simulink model "alu"  (R2022b)
settings: Solver=VariableStepAuto  StartTime=0.0  StopTime=10.0  RelTol=1e-3
settings Model: Creator=F1  LastModifiedBy=Namratha
settings SolverCC: AlgebraicLoopSolver=TrustRegion
settings DebuggingCC: UnconnectedInputMsg=warning  UnconnectedOutputMsg=warning  UnconnectedLineMsg=warning  SFMachineParentedDataDiag=warning
settings ModelReferenceCC: EnableRefExpFcnMdlSchedulingChecks=on

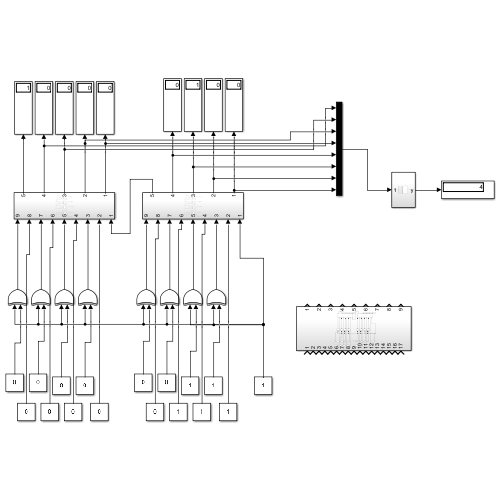
[thumbnail: Simulink's stored preview of the top-level diagram]
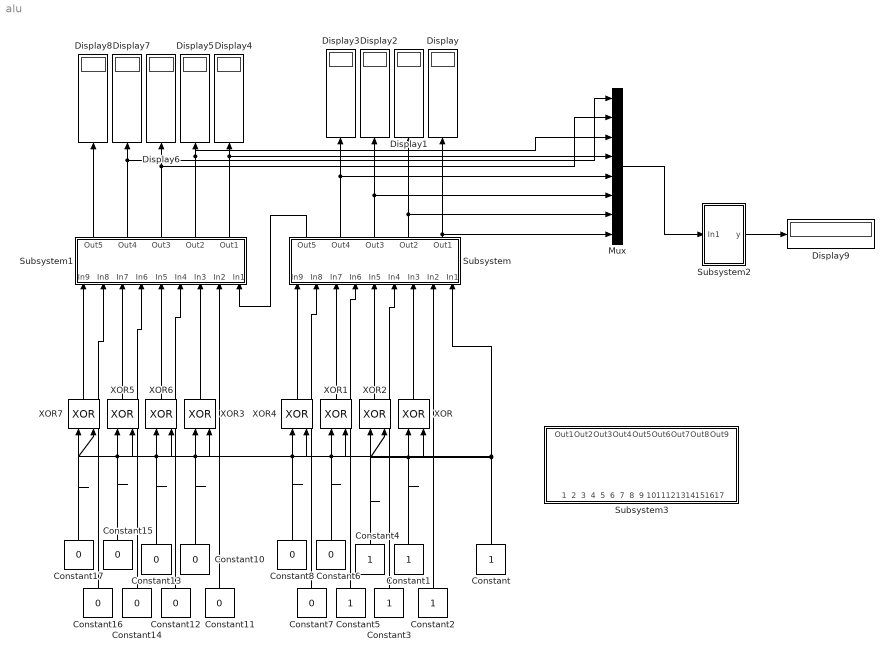
== system alu ==
  Constant{,1..5} (6 alike) : Constant
  Constant{6..8,10..17} (11 alike) : Constant  Value=0
  Display{,1..9} (10 alike) : Display
  Mux : Mux  Inputs=8
  Subsystem : Subsystem
  Subsystem1 : Subsystem
  Subsystem2 : Subsystem
  Subsystem3 : Subsystem
  XOR{,1..7} (8 alike) : Logic  Operator=XOR  IconShape=distinctive  AllPortsSameDT=off  OutDataTypeStr=boolean
  wires:
  XOR/1 -> Subsystem/3(In3)
  XOR2/1 -> Subsystem/5(In5)
  XOR1/1 -> Subsystem/7(In7)
  XOR4/1 -> Subsystem/9(In9)
  Constant1/1 -> XOR/2
  Constant2/1 -> Subsystem/2(In2)
  Constant3/1 -> Subsystem/4(In4)
  Constant4/1 -> XOR2/2
  Constant5/1 -> Subsystem/6(In6)
  Constant6/1 -> XOR1/2
  Constant7/1 -> Subsystem/8(In8)
  Constant8/1 -> XOR4/2
  Constant12/1 -> Subsystem1/4(In4)
  Constant15/1 -> XOR5/2
  XOR3/1 -> Subsystem1/3(In3)
  Constant/1 -> XOR2/1, XOR/1, XOR5/1, XOR7/1, XOR6/1, XOR3/1, XOR4/1, XOR1/1, Subsystem/1(In1)
  Constant13/1 -> XOR6/2
  Constant11/1 -> Subsystem1/2(In2)
  Constant16/1 -> Subsystem1/8(In8)
  Constant10/1 -> XOR3/2
  XOR7/1 -> Subsystem1/9(In9)
  XOR6/1 -> Subsystem1/5(In5)
  Constant17/1 -> XOR7/2
  XOR5/1 -> Subsystem1/7(In7)
  Constant14/1 -> Subsystem1/6(In6)
  Subsystem/5(Out5) -> Subsystem1/1(In1)
  Subsystem/1(Out1) -> Display/1, Mux/8
  Subsystem/2(Out2) -> Display1/1, Mux/7
  Subsystem/3(Out3) -> Display2/1, Mux/6
  Subsystem/4(Out4) -> Display3/1, Mux/5
  Subsystem1/1(Out1) -> Mux/4, Display4/1
  Subsystem1/2(Out2) -> Mux/3, Display5/1
  Subsystem1/3(Out3) -> Display6/1, Mux/2
  Subsystem1/4(Out4) -> Display7/1, Mux/1
  Subsystem1/5(Out5) -> Display8/1
  Mux/1 -> Subsystem2/1(In1)
  Subsystem2/1(y) -> Display9/1

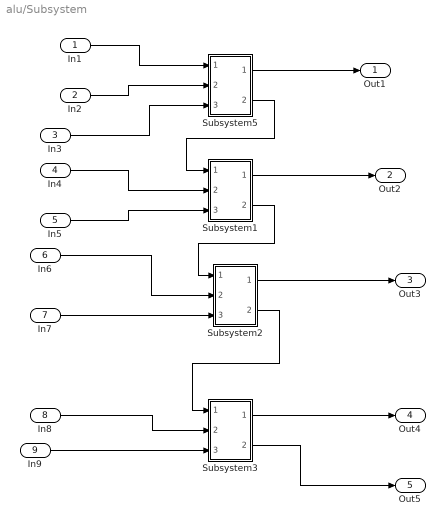
== system alu/Subsystem ==
  In1 : Inport
  In2 : Inport  Port=2
  In3 : Inport  Port=3
  In4 : Inport  Port=4
  In5 : Inport  Port=5
  In6 : Inport  Port=6
  In7 : Inport  Port=7
  In8 : Inport  Port=8
  In9 : Inport  Port=9
  Subsystem1 : Subsystem
  Subsystem2 : Subsystem
  Subsystem3 : Subsystem
  Subsystem5 : Subsystem
  Out1 : Outport
  Out2 : Outport  Port=2
  Out3 : Outport  Port=3
  Out4 : Outport  Port=4
  Out5 : Outport  Port=5
  wires:
  Subsystem2/2(Out2) -> Subsystem3/1(In1)
  In8/1 -> Subsystem3/2(In2)
  Subsystem5/2(Out2) -> Subsystem1/1(In1)
  Subsystem2/1(Out1) -> Out3/1
  Subsystem1/2(Out2) -> Subsystem2/1(In1)
  In6/1 -> Subsystem2/2(In2)
  In7/1 -> Subsystem2/3(In3)
  In4/1 -> Subsystem1/2(In2)
  Subsystem3/1(Out1) -> Out4/1
  In9/1 -> Subsystem3/3(In3)
  In2/1 -> Subsystem5/2(In2)
  In3/1 -> Subsystem5/3(In3)
  In1/1 -> Subsystem5/1(In1)
  Subsystem5/1(Out1) -> Out1/1
  Subsystem3/2(Out2) -> Out5/1
  Subsystem1/1(Out1) -> Out2/1
  In5/1 -> Subsystem1/3(In3)

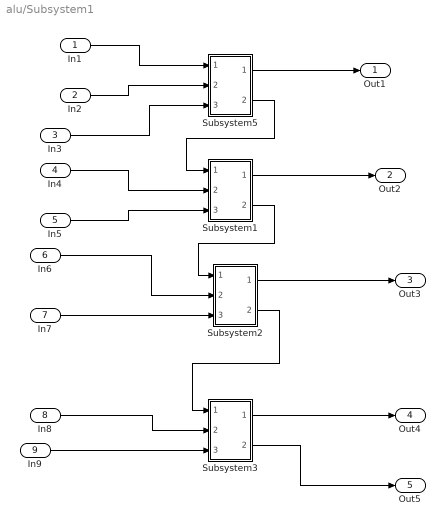
== system alu/Subsystem1 ==
  In1 : Inport
  In2 : Inport  Port=2
  In3 : Inport  Port=3
  In4 : Inport  Port=4
  In5 : Inport  Port=5
  In6 : Inport  Port=6
  In7 : Inport  Port=7
  In8 : Inport  Port=8
  In9 : Inport  Port=9
  Subsystem1 : Subsystem
  Subsystem2 : Subsystem
  Subsystem3 : Subsystem
  Subsystem5 : Subsystem
  Out1 : Outport
  Out2 : Outport  Port=2
  Out3 : Outport  Port=3
  Out4 : Outport  Port=4
  Out5 : Outport  Port=5
  wires:
  Subsystem2/2(Out2) -> Subsystem3/1(In1)
  In8/1 -> Subsystem3/2(In2)
  Subsystem5/2(Out2) -> Subsystem1/1(In1)
  Subsystem2/1(Out1) -> Out3/1
  Subsystem1/2(Out2) -> Subsystem2/1(In1)
  In6/1 -> Subsystem2/2(In2)
  In7/1 -> Subsystem2/3(In3)
  In4/1 -> Subsystem1/2(In2)
  Subsystem3/1(Out1) -> Out4/1
  In9/1 -> Subsystem3/3(In3)
  In2/1 -> Subsystem5/2(In2)
  In3/1 -> Subsystem5/3(In3)
  In1/1 -> Subsystem5/1(In1)
  Subsystem5/1(Out1) -> Out1/1
  Subsystem3/2(Out2) -> Out5/1
  Subsystem1/1(Out1) -> Out2/1
  In5/1 -> Subsystem1/3(In3)

== system alu/Subsystem2 ==
  In1 : Inport
  Demux : Demux  Outputs=8
  MATLAB Function : MATLAB Function  TreatAsAtomicUnit=on
  y : Outport
  wires:
  Demux/8 -> MATLAB Function/8(b0)
  Demux/2 -> MATLAB Function/2(b6)
  MATLAB Function/1(y) -> y/1
  Demux/7 -> MATLAB Function/7(b1)
  Demux/4 -> MATLAB Function/4(b4)
  Demux/6 -> MATLAB Function/6(b2)
  Demux/3 -> MATLAB Function/3(b5)
  Demux/1 -> MATLAB Function/1(b7)
  Demux/5 -> MATLAB Function/5(b3)
  In1/1 -> Demux/1

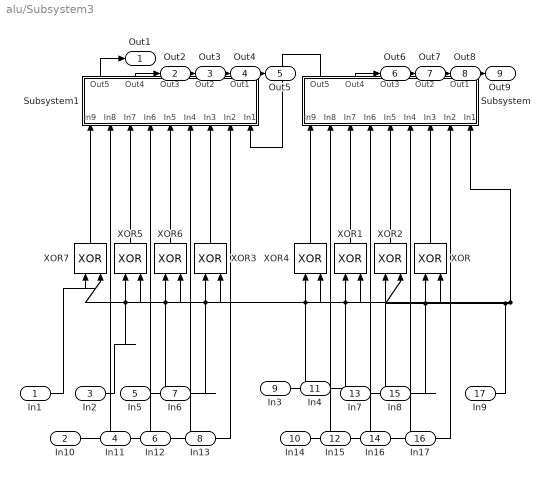
== system alu/Subsystem3 ==
  In1 : Inport
  In10 : Inport  Port=2
  In2 : Inport  Port=3
  In11 : Inport  Port=4
  In5 : Inport  Port=5
  In12 : Inport  Port=6
  In6 : Inport  Port=7
  In13 : Inport  Port=8
  In3 : Inport  Port=9
  In14 : Inport  Port=10
  In4 : Inport  Port=11
  In15 : Inport  Port=12
  In7 : Inport  Port=13
  In16 : Inport  Port=14
  In8 : Inport  Port=15
  In17 : Inport  Port=16
  In9 : Inport  Port=17
  Subsystem : Subsystem
  Subsystem1 : Subsystem
  XOR{,1..7} (8 alike) : Logic  Operator=XOR  IconShape=distinctive  AllPortsSameDT=off  OutDataTypeStr=boolean
  Out1 : Outport
  Out2 : Outport  Port=2
  Out3 : Outport  Port=3
  Out4 : Outport  Port=4
  Out5 : Outport  Port=5
  Out6 : Outport  Port=6
  Out7 : Outport  Port=7
  Out8 : Outport  Port=8
  Out9 : Outport  Port=9
  wires:
  In1/1 -> XOR7/2
  XOR3/1 -> Subsystem1/3(In3)
  In17/1 -> Subsystem/2(In2)
  In9/1 -> XOR5/1, XOR7/1, XOR6/1, XOR3/1, XOR4/1, XOR1/1, Subsystem/1(In1), XOR2/1, XOR/1
  Subsystem1/3(Out3) -> Out3/1
  In3/1 -> XOR4/2
  XOR1/1 -> Subsystem/7(In7)
  Subsystem1/1(Out1) -> Out5/1
  In16/1 -> Subsystem/4(In4)
  In15/1 -> Subsystem/6(In6)
  XOR6/1 -> Subsystem1/5(In5)
  XOR2/1 -> Subsystem/5(In5)
  In13/1 -> Subsystem1/2(In2)
  Subsystem/2(Out2) -> Out8/1
  In6/1 -> XOR3/2
  Subsystem/5(Out5) -> Subsystem1/1(In1)
  Subsystem/3(Out3) -> Out7/1
  In2/1 -> XOR5/2
  Subsystem1/5(Out5) -> Out1/1
  XOR5/1 -> Subsystem1/7(In7)
  XOR4/1 -> Subsystem/9(In9)
  XOR7/1 -> Subsystem1/9(In9)
  In8/1 -> XOR/2
  XOR/1 -> Subsystem/3(In3)
  Subsystem/4(Out4) -> Out6/1
  In7/1 -> XOR2/2
  In11/1 -> Subsystem1/6(In6)
  In10/1 -> Subsystem1/8(In8)
  In5/1 -> XOR6/2
  In14/1 -> Subsystem/8(In8)
  In4/1 -> XOR1/2
  In12/1 -> Subsystem1/4(In4)
  Subsystem1/4(Out4) -> Out2/1
  Subsystem1/2(Out2) -> Out4/1
  Subsystem/1(Out1) -> Out9/1

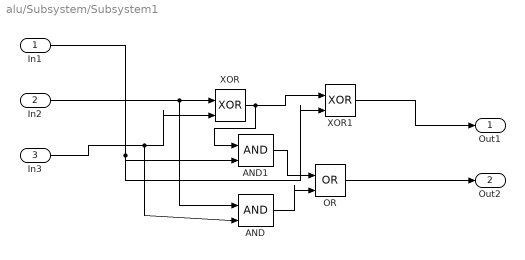
== system alu/Subsystem/Subsystem1 ==
  In1 : Inport
  In2 : Inport  Port=2
  In3 : Inport  Port=3
  AND : Logic  IconShape=distinctive  AllPortsSameDT=off  OutDataTypeStr=boolean
  AND1 : Logic  IconShape=distinctive  AllPortsSameDT=off  OutDataTypeStr=boolean
  OR : Logic  Operator=OR  IconShape=distinctive  AllPortsSameDT=off  OutDataTypeStr=boolean
  XOR : Logic  Operator=XOR  IconShape=distinctive  AllPortsSameDT=off  OutDataTypeStr=boolean
  XOR1 : Logic  Operator=XOR  IconShape=distinctive  AllPortsSameDT=off  OutDataTypeStr=boolean
  Out1 : Outport
  Out2 : Outport  Port=2
  wires:
  AND1/1 -> OR/1
  AND/1 -> OR/2
  In3/1 -> AND/2, XOR/2
  In2/1 -> AND/1, XOR/1
  In1/1 -> XOR1/2, AND1/2
  XOR/1 -> AND1/1, XOR1/1
  XOR1/1 -> Out1/1
  OR/1 -> Out2/1

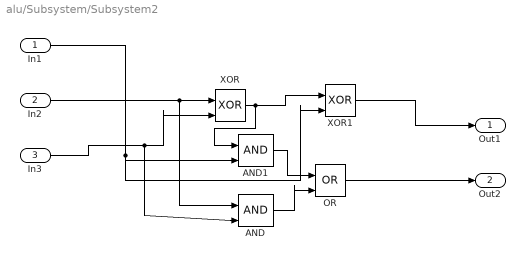
== system alu/Subsystem/Subsystem2 ==
  In1 : Inport
  In2 : Inport  Port=2
  In3 : Inport  Port=3
  AND : Logic  IconShape=distinctive  AllPortsSameDT=off  OutDataTypeStr=boolean
  AND1 : Logic  IconShape=distinctive  AllPortsSameDT=off  OutDataTypeStr=boolean
  OR : Logic  Operator=OR  IconShape=distinctive  AllPortsSameDT=off  OutDataTypeStr=boolean
  XOR : Logic  Operator=XOR  IconShape=distinctive  AllPortsSameDT=off  OutDataTypeStr=boolean
  XOR1 : Logic  Operator=XOR  IconShape=distinctive  AllPortsSameDT=off  OutDataTypeStr=boolean
  Out1 : Outport
  Out2 : Outport  Port=2
  wires:
  AND1/1 -> OR/1
  AND/1 -> OR/2
  In3/1 -> AND/2, XOR/2
  In2/1 -> AND/1, XOR/1
  In1/1 -> XOR1/2, AND1/2
  XOR/1 -> AND1/1, XOR1/1
  XOR1/1 -> Out1/1
  OR/1 -> Out2/1

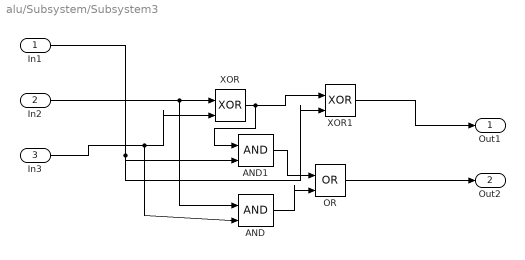
== system alu/Subsystem/Subsystem3 ==
  In1 : Inport
  In2 : Inport  Port=2
  In3 : Inport  Port=3
  AND : Logic  IconShape=distinctive  AllPortsSameDT=off  OutDataTypeStr=boolean
  AND1 : Logic  IconShape=distinctive  AllPortsSameDT=off  OutDataTypeStr=boolean
  OR : Logic  Operator=OR  IconShape=distinctive  AllPortsSameDT=off  OutDataTypeStr=boolean
  XOR : Logic  Operator=XOR  IconShape=distinctive  AllPortsSameDT=off  OutDataTypeStr=boolean
  XOR1 : Logic  Operator=XOR  IconShape=distinctive  AllPortsSameDT=off  OutDataTypeStr=boolean
  Out1 : Outport
  Out2 : Outport  Port=2
  wires:
  AND1/1 -> OR/1
  AND/1 -> OR/2
  In3/1 -> AND/2, XOR/2
  In2/1 -> AND/1, XOR/1
  In1/1 -> XOR1/2, AND1/2
  XOR/1 -> AND1/1, XOR1/1
  XOR1/1 -> Out1/1
  OR/1 -> Out2/1

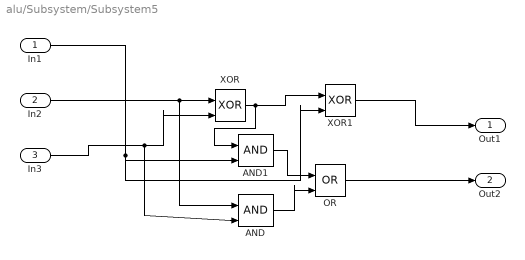
== system alu/Subsystem/Subsystem5 ==
  In1 : Inport
  In2 : Inport  Port=2
  In3 : Inport  Port=3
  AND : Logic  IconShape=distinctive  AllPortsSameDT=off  OutDataTypeStr=boolean
  AND1 : Logic  IconShape=distinctive  AllPortsSameDT=off  OutDataTypeStr=boolean
  OR : Logic  Operator=OR  IconShape=distinctive  AllPortsSameDT=off  OutDataTypeStr=boolean
  XOR : Logic  Operator=XOR  IconShape=distinctive  AllPortsSameDT=off  OutDataTypeStr=boolean
  XOR1 : Logic  Operator=XOR  IconShape=distinctive  AllPortsSameDT=off  OutDataTypeStr=boolean
  Out1 : Outport
  Out2 : Outport  Port=2
  wires:
  AND1/1 -> OR/1
  AND/1 -> OR/2
  In3/1 -> AND/2, XOR/2
  In2/1 -> AND/1, XOR/1
  In1/1 -> XOR1/2, AND1/2
  XOR/1 -> AND1/1, XOR1/1
  XOR1/1 -> Out1/1
  OR/1 -> Out2/1

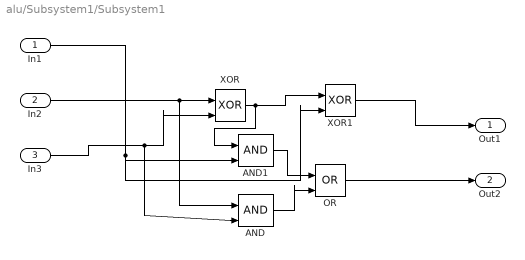
== system alu/Subsystem1/Subsystem1 ==
  In1 : Inport
  In2 : Inport  Port=2
  In3 : Inport  Port=3
  AND : Logic  IconShape=distinctive  AllPortsSameDT=off  OutDataTypeStr=boolean
  AND1 : Logic  IconShape=distinctive  AllPortsSameDT=off  OutDataTypeStr=boolean
  OR : Logic  Operator=OR  IconShape=distinctive  AllPortsSameDT=off  OutDataTypeStr=boolean
  XOR : Logic  Operator=XOR  IconShape=distinctive  AllPortsSameDT=off  OutDataTypeStr=boolean
  XOR1 : Logic  Operator=XOR  IconShape=distinctive  AllPortsSameDT=off  OutDataTypeStr=boolean
  Out1 : Outport
  Out2 : Outport  Port=2
  wires:
  AND1/1 -> OR/1
  AND/1 -> OR/2
  In3/1 -> AND/2, XOR/2
  In2/1 -> AND/1, XOR/1
  In1/1 -> XOR1/2, AND1/2
  XOR/1 -> AND1/1, XOR1/1
  XOR1/1 -> Out1/1
  OR/1 -> Out2/1

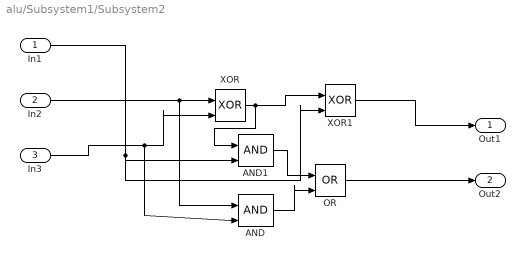
== system alu/Subsystem1/Subsystem2 ==
  In1 : Inport
  In2 : Inport  Port=2
  In3 : Inport  Port=3
  AND : Logic  IconShape=distinctive  AllPortsSameDT=off  OutDataTypeStr=boolean
  AND1 : Logic  IconShape=distinctive  AllPortsSameDT=off  OutDataTypeStr=boolean
  OR : Logic  Operator=OR  IconShape=distinctive  AllPortsSameDT=off  OutDataTypeStr=boolean
  XOR : Logic  Operator=XOR  IconShape=distinctive  AllPortsSameDT=off  OutDataTypeStr=boolean
  XOR1 : Logic  Operator=XOR  IconShape=distinctive  AllPortsSameDT=off  OutDataTypeStr=boolean
  Out1 : Outport
  Out2 : Outport  Port=2
  wires:
  AND1/1 -> OR/1
  AND/1 -> OR/2
  In3/1 -> AND/2, XOR/2
  In2/1 -> AND/1, XOR/1
  In1/1 -> XOR1/2, AND1/2
  XOR/1 -> AND1/1, XOR1/1
  XOR1/1 -> Out1/1
  OR/1 -> Out2/1

== system alu/Subsystem1/Subsystem3 ==
  In1 : Inport
  In2 : Inport  Port=2
  In3 : Inport  Port=3
  AND : Logic  IconShape=distinctive  AllPortsSameDT=off  OutDataTypeStr=boolean
  AND1 : Logic  IconShape=distinctive  AllPortsSameDT=off  OutDataTypeStr=boolean
  OR : Logic  Operator=OR  IconShape=distinctive  AllPortsSameDT=off  OutDataTypeStr=boolean
  XOR : Logic  Operator=XOR  IconShape=distinctive  AllPortsSameDT=off  OutDataTypeStr=boolean
  XOR1 : Logic  Operator=XOR  IconShape=distinctive  AllPortsSameDT=off  OutDataTypeStr=boolean
  Out1 : Outport
  Out2 : Outport  Port=2
  wires:
  AND1/1 -> OR/1
  AND/1 -> OR/2
  In3/1 -> AND/2, XOR/2
  In2/1 -> AND/1, XOR/1
  In1/1 -> XOR1/2, AND1/2
  XOR/1 -> AND1/1, XOR1/1
  XOR1/1 -> Out1/1
  OR/1 -> Out2/1

== system alu/Subsystem1/Subsystem5 ==
  In1 : Inport
  In2 : Inport  Port=2
  In3 : Inport  Port=3
  AND : Logic  IconShape=distinctive  AllPortsSameDT=off  OutDataTypeStr=boolean
  AND1 : Logic  IconShape=distinctive  AllPortsSameDT=off  OutDataTypeStr=boolean
  OR : Logic  Operator=OR  IconShape=distinctive  AllPortsSameDT=off  OutDataTypeStr=boolean
  XOR : Logic  Operator=XOR  IconShape=distinctive  AllPortsSameDT=off  OutDataTypeStr=boolean
  XOR1 : Logic  Operator=XOR  IconShape=distinctive  AllPortsSameDT=off  OutDataTypeStr=boolean
  Out1 : Outport
  Out2 : Outport  Port=2
  wires:
  AND1/1 -> OR/1
  AND/1 -> OR/2
  In3/1 -> AND/2, XOR/2
  In2/1 -> AND/1, XOR/1
  In1/1 -> XOR1/2, AND1/2
  XOR/1 -> AND1/1, XOR1/1
  XOR1/1 -> Out1/1
  OR/1 -> Out2/1

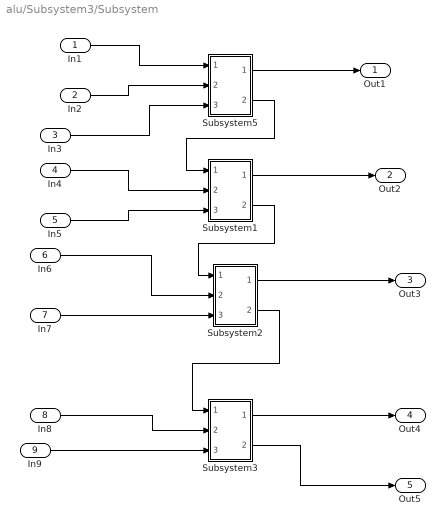
== system alu/Subsystem3/Subsystem ==
  In1 : Inport
  In2 : Inport  Port=2
  In3 : Inport  Port=3
  In4 : Inport  Port=4
  In5 : Inport  Port=5
  In6 : Inport  Port=6
  In7 : Inport  Port=7
  In8 : Inport  Port=8
  In9 : Inport  Port=9
  Subsystem1 : Subsystem
  Subsystem2 : Subsystem
  Subsystem3 : Subsystem
  Subsystem5 : Subsystem
  Out1 : Outport
  Out2 : Outport  Port=2
  Out3 : Outport  Port=3
  Out4 : Outport  Port=4
  Out5 : Outport  Port=5
  wires:
  Subsystem2/2(Out2) -> Subsystem3/1(In1)
  In8/1 -> Subsystem3/2(In2)
  Subsystem5/2(Out2) -> Subsystem1/1(In1)
  Subsystem2/1(Out1) -> Out3/1
  Subsystem1/2(Out2) -> Subsystem2/1(In1)
  In6/1 -> Subsystem2/2(In2)
  In7/1 -> Subsystem2/3(In3)
  In4/1 -> Subsystem1/2(In2)
  Subsystem3/1(Out1) -> Out4/1
  In9/1 -> Subsystem3/3(In3)
  In2/1 -> Subsystem5/2(In2)
  In3/1 -> Subsystem5/3(In3)
  In1/1 -> Subsystem5/1(In1)
  Subsystem5/1(Out1) -> Out1/1
  Subsystem3/2(Out2) -> Out5/1
  Subsystem1/1(Out1) -> Out2/1
  In5/1 -> Subsystem1/3(In3)

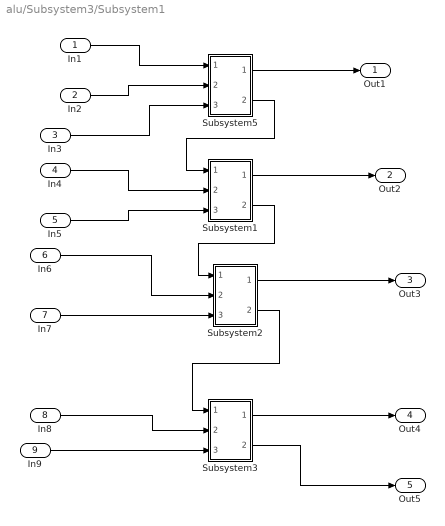
== system alu/Subsystem3/Subsystem1 ==
  In1 : Inport
  In2 : Inport  Port=2
  In3 : Inport  Port=3
  In4 : Inport  Port=4
  In5 : Inport  Port=5
  In6 : Inport  Port=6
  In7 : Inport  Port=7
  In8 : Inport  Port=8
  In9 : Inport  Port=9
  Subsystem1 : Subsystem
  Subsystem2 : Subsystem
  Subsystem3 : Subsystem
  Subsystem5 : Subsystem
  Out1 : Outport
  Out2 : Outport  Port=2
  Out3 : Outport  Port=3
  Out4 : Outport  Port=4
  Out5 : Outport  Port=5
  wires:
  Subsystem2/2(Out2) -> Subsystem3/1(In1)
  In8/1 -> Subsystem3/2(In2)
  Subsystem5/2(Out2) -> Subsystem1/1(In1)
  Subsystem2/1(Out1) -> Out3/1
  Subsystem1/2(Out2) -> Subsystem2/1(In1)
  In6/1 -> Subsystem2/2(In2)
  In7/1 -> Subsystem2/3(In3)
  In4/1 -> Subsystem1/2(In2)
  Subsystem3/1(Out1) -> Out4/1
  In9/1 -> Subsystem3/3(In3)
  In2/1 -> Subsystem5/2(In2)
  In3/1 -> Subsystem5/3(In3)
  In1/1 -> Subsystem5/1(In1)
  Subsystem5/1(Out1) -> Out1/1
  Subsystem3/2(Out2) -> Out5/1
  Subsystem1/1(Out1) -> Out2/1
  In5/1 -> Subsystem1/3(In3)

== system alu/Subsystem3/Subsystem/Subsystem1 ==
  In1 : Inport
  In2 : Inport  Port=2
  In3 : Inport  Port=3
  AND : Logic  IconShape=distinctive  AllPortsSameDT=off  OutDataTypeStr=boolean
  AND1 : Logic  IconShape=distinctive  AllPortsSameDT=off  OutDataTypeStr=boolean
  OR : Logic  Operator=OR  IconShape=distinctive  AllPortsSameDT=off  OutDataTypeStr=boolean
  XOR : Logic  Operator=XOR  IconShape=distinctive  AllPortsSameDT=off  OutDataTypeStr=boolean
  XOR1 : Logic  Operator=XOR  IconShape=distinctive  AllPortsSameDT=off  OutDataTypeStr=boolean
  Out1 : Outport
  Out2 : Outport  Port=2
  wires:
  AND1/1 -> OR/1
  AND/1 -> OR/2
  In3/1 -> AND/2, XOR/2
  In2/1 -> AND/1, XOR/1
  In1/1 -> XOR1/2, AND1/2
  XOR/1 -> AND1/1, XOR1/1
  XOR1/1 -> Out1/1
  OR/1 -> Out2/1

== system alu/Subsystem3/Subsystem/Subsystem2 ==
  In1 : Inport
  In2 : Inport  Port=2
  In3 : Inport  Port=3
  AND : Logic  IconShape=distinctive  AllPortsSameDT=off  OutDataTypeStr=boolean
  AND1 : Logic  IconShape=distinctive  AllPortsSameDT=off  OutDataTypeStr=boolean
  OR : Logic  Operator=OR  IconShape=distinctive  AllPortsSameDT=off  OutDataTypeStr=boolean
  XOR : Logic  Operator=XOR  IconShape=distinctive  AllPortsSameDT=off  OutDataTypeStr=boolean
  XOR1 : Logic  Operator=XOR  IconShape=distinctive  AllPortsSameDT=off  OutDataTypeStr=boolean
  Out1 : Outport
  Out2 : Outport  Port=2
  wires:
  AND1/1 -> OR/1
  AND/1 -> OR/2
  In3/1 -> AND/2, XOR/2
  In2/1 -> AND/1, XOR/1
  In1/1 -> XOR1/2, AND1/2
  XOR/1 -> AND1/1, XOR1/1
  XOR1/1 -> Out1/1
  OR/1 -> Out2/1

== system alu/Subsystem3/Subsystem/Subsystem3 ==
  In1 : Inport
  In2 : Inport  Port=2
  In3 : Inport  Port=3
  AND : Logic  IconShape=distinctive  AllPortsSameDT=off  OutDataTypeStr=boolean
  AND1 : Logic  IconShape=distinctive  AllPortsSameDT=off  OutDataTypeStr=boolean
  OR : Logic  Operator=OR  IconShape=distinctive  AllPortsSameDT=off  OutDataTypeStr=boolean
  XOR : Logic  Operator=XOR  IconShape=distinctive  AllPortsSameDT=off  OutDataTypeStr=boolean
  XOR1 : Logic  Operator=XOR  IconShape=distinctive  AllPortsSameDT=off  OutDataTypeStr=boolean
  Out1 : Outport
  Out2 : Outport  Port=2
  wires:
  AND1/1 -> OR/1
  AND/1 -> OR/2
  In3/1 -> AND/2, XOR/2
  In2/1 -> AND/1, XOR/1
  In1/1 -> XOR1/2, AND1/2
  XOR/1 -> AND1/1, XOR1/1
  XOR1/1 -> Out1/1
  OR/1 -> Out2/1

== system alu/Subsystem3/Subsystem/Subsystem5 ==
  In1 : Inport
  In2 : Inport  Port=2
  In3 : Inport  Port=3
  AND : Logic  IconShape=distinctive  AllPortsSameDT=off  OutDataTypeStr=boolean
  AND1 : Logic  IconShape=distinctive  AllPortsSameDT=off  OutDataTypeStr=boolean
  OR : Logic  Operator=OR  IconShape=distinctive  AllPortsSameDT=off  OutDataTypeStr=boolean
  XOR : Logic  Operator=XOR  IconShape=distinctive  AllPortsSameDT=off  OutDataTypeStr=boolean
  XOR1 : Logic  Operator=XOR  IconShape=distinctive  AllPortsSameDT=off  OutDataTypeStr=boolean
  Out1 : Outport
  Out2 : Outport  Port=2
  wires:
  AND1/1 -> OR/1
  AND/1 -> OR/2
  In3/1 -> AND/2, XOR/2
  In2/1 -> AND/1, XOR/1
  In1/1 -> XOR1/2, AND1/2
  XOR/1 -> AND1/1, XOR1/1
  XOR1/1 -> Out1/1
  OR/1 -> Out2/1

== system alu/Subsystem3/Subsystem1/Subsystem1 ==
  In1 : Inport
  In2 : Inport  Port=2
  In3 : Inport  Port=3
  AND : Logic  IconShape=distinctive  AllPortsSameDT=off  OutDataTypeStr=boolean
  AND1 : Logic  IconShape=distinctive  AllPortsSameDT=off  OutDataTypeStr=boolean
  OR : Logic  Operator=OR  IconShape=distinctive  AllPortsSameDT=off  OutDataTypeStr=boolean
  XOR : Logic  Operator=XOR  IconShape=distinctive  AllPortsSameDT=off  OutDataTypeStr=boolean
  XOR1 : Logic  Operator=XOR  IconShape=distinctive  AllPortsSameDT=off  OutDataTypeStr=boolean
  Out1 : Outport
  Out2 : Outport  Port=2
  wires:
  AND1/1 -> OR/1
  AND/1 -> OR/2
  In3/1 -> AND/2, XOR/2
  In2/1 -> AND/1, XOR/1
  In1/1 -> XOR1/2, AND1/2
  XOR/1 -> AND1/1, XOR1/1
  XOR1/1 -> Out1/1
  OR/1 -> Out2/1

== system alu/Subsystem3/Subsystem1/Subsystem2 ==
  In1 : Inport
  In2 : Inport  Port=2
  In3 : Inport  Port=3
  AND : Logic  IconShape=distinctive  AllPortsSameDT=off  OutDataTypeStr=boolean
  AND1 : Logic  IconShape=distinctive  AllPortsSameDT=off  OutDataTypeStr=boolean
  OR : Logic  Operator=OR  IconShape=distinctive  AllPortsSameDT=off  OutDataTypeStr=boolean
  XOR : Logic  Operator=XOR  IconShape=distinctive  AllPortsSameDT=off  OutDataTypeStr=boolean
  XOR1 : Logic  Operator=XOR  IconShape=distinctive  AllPortsSameDT=off  OutDataTypeStr=boolean
  Out1 : Outport
  Out2 : Outport  Port=2
  wires:
  AND1/1 -> OR/1
  AND/1 -> OR/2
  In3/1 -> AND/2, XOR/2
  In2/1 -> AND/1, XOR/1
  In1/1 -> XOR1/2, AND1/2
  XOR/1 -> AND1/1, XOR1/1
  XOR1/1 -> Out1/1
  OR/1 -> Out2/1

== system alu/Subsystem3/Subsystem1/Subsystem3 ==
  In1 : Inport
  In2 : Inport  Port=2
  In3 : Inport  Port=3
  AND : Logic  IconShape=distinctive  AllPortsSameDT=off  OutDataTypeStr=boolean
  AND1 : Logic  IconShape=distinctive  AllPortsSameDT=off  OutDataTypeStr=boolean
  OR : Logic  Operator=OR  IconShape=distinctive  AllPortsSameDT=off  OutDataTypeStr=boolean
  XOR : Logic  Operator=XOR  IconShape=distinctive  AllPortsSameDT=off  OutDataTypeStr=boolean
  XOR1 : Logic  Operator=XOR  IconShape=distinctive  AllPortsSameDT=off  OutDataTypeStr=boolean
  Out1 : Outport
  Out2 : Outport  Port=2
  wires:
  AND1/1 -> OR/1
  AND/1 -> OR/2
  In3/1 -> AND/2, XOR/2
  In2/1 -> AND/1, XOR/1
  In1/1 -> XOR1/2, AND1/2
  XOR/1 -> AND1/1, XOR1/1
  XOR1/1 -> Out1/1
  OR/1 -> Out2/1

== system alu/Subsystem3/Subsystem1/Subsystem5 ==
  In1 : Inport
  In2 : Inport  Port=2
  In3 : Inport  Port=3
  AND : Logic  IconShape=distinctive  AllPortsSameDT=off  OutDataTypeStr=boolean
  AND1 : Logic  IconShape=distinctive  AllPortsSameDT=off  OutDataTypeStr=boolean
  OR : Logic  Operator=OR  IconShape=distinctive  AllPortsSameDT=off  OutDataTypeStr=boolean
  XOR : Logic  Operator=XOR  IconShape=distinctive  AllPortsSameDT=off  OutDataTypeStr=boolean
  XOR1 : Logic  Operator=XOR  IconShape=distinctive  AllPortsSameDT=off  OutDataTypeStr=boolean
  Out1 : Outport
  Out2 : Outport  Port=2
  wires:
  AND1/1 -> OR/1
  AND/1 -> OR/2
  In3/1 -> AND/2, XOR/2
  In2/1 -> AND/1, XOR/1
  In1/1 -> XOR1/2, AND1/2
  XOR/1 -> AND1/1, XOR1/1
  XOR1/1 -> Out1/1
  OR/1 -> Out2/1

== matlab function alu/Subsystem2/MATLAB Function ==
  data: b7 input; y output [0..255]; b6 input; b5 input; b4 input; b3 input; b2 input; b1 input; b0 input
function y = fcn(b7   , b6  , b5   , b4  , b3   , b2   , b1    , b0    )
y = b7*2^7 + b6*2^6 + b5*2^5 + b4*2^4 + b3*2^3 + b2*2^2 + b1*2^1 + b0*2^0 ;
end



%str_x = sprintf("%i",u);
% remove the spaces in the string, so it 
% becomes '10000000'
%str_x(isspace(str_x)) = '';
% now use BIN2DEC to convert the binary 
% string to a decimal number
%y = bin2dec(str_x);
%y = class(u);
%y = bin2dec(sprintf('%d',u));
